simulink model "pro4"  (R2020a)
settings: Solver=VariableStepAuto  StartTime=0.0  StopTime=10.0  RelTol=1e-3
libraries: simulink x1
settings Model: Creator=aa  LastModifiedBy=aa

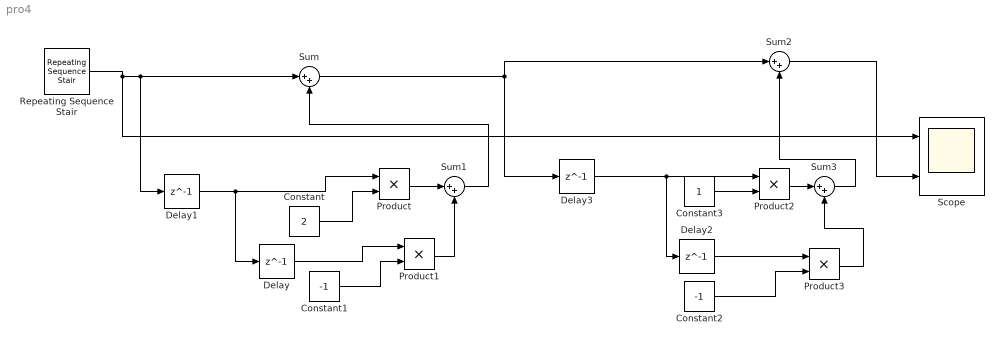
== system pro4 ==
  Constant : Constant  Value=2
  Constant1 : Constant  Value=-1
  Constant2 : Constant  Value=-1
  Constant3 : Constant
  Delay{,1..3} (4 alike) : Delay  DelayLength=1
  Product{,1..3} (4 alike) : Product
  Repeating Sequence Stair : simulink/Sources/Repeating Sequence Stair  OutValues=[1 0 0 0 0 0 0 ].'  tsamp=-1  OutMin=[]  OutMax=[]  OutDataTypeStr=double  OutputDataTypeScalingMode=double  OutDataType=fixdt(0,8)  ConRadixGroup=Best Precision: Vector-wise  OutScaling=2^-12
  Scope : Scope  NumInputPorts=2
  Sum{,1..3} (4 alike) : Sum  Inputs=|++
  wires:
  Product3/1 -> Sum3/2
  Constant2/1 -> Product3/2
  Sum3/1 -> Sum2/2
  Sum2/1 -> Scope/2
  Constant1/1 -> Product1/2
  Delay2/1 -> Product3/1
  Repeating Sequence Stair/1 -> Scope/1, Sum/1, Delay1/1
  Sum1/1 -> Sum/2
  Constant3/1 -> Product2/2
  Product/1 -> Sum1/1
  Sum/1 -> Delay3/1, Sum2/1
  Product1/1 -> Sum1/2
  Delay3/1 -> Delay2/1, Product2/1
  Product2/1 -> Sum3/1
  Delay/1 -> Product1/1
  Constant/1 -> Product/2
  Delay1/1 -> Product/1, Delay/1
